simulink subsystem "PipeModule"  (R2021b)
settings: Solver=VariableStepAuto  StartTime=0.0  StopTime=10.0  RelTol=1e-3
libraries: SimscapeFluids_lib x1
settings Model: Creator=silen  LastModifiedBy=silen

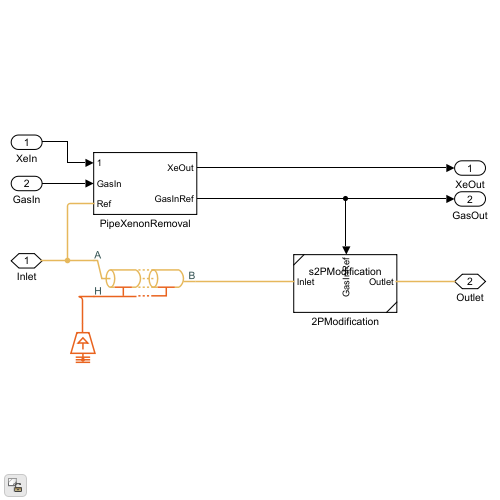
[thumbnail: Simulink's stored preview of the top-level diagram]
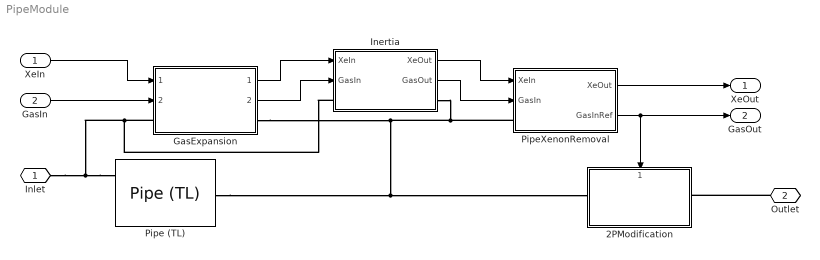
== system PipeModule ==
  XeIn : Inport
  GasIn : Inport  Port=2
  2PModification : Subsystem  ReferencedSubsystem=s2PModification
      settings: PortSchema="{\"entries\":[{\"content\":{\"sides\":[{\"content\":{\"connectorIds\":[\"LConn1\"]},\"type\":\"ConnectorPlacement.EquallySpacedRectSide\",\"uuid\":\"411e3aad-085a-4802-ae1a-063314444375\"},{\"content\":{\"connectorIds\":[\"RConn1\"],\"side\":\"RIGHT\"},\"type\":\"ConnectorPlacement.EquallySpacedRectSide\",\"uuid\":\"fb5502b3-1e9f-42df-a026-3213f778497c\"},{\"content\":{\"connectorIds\":[\"In1\"],\"side\":\"TOP\"},\"type\":\"ConnectorPlacement.EquallySpacedRectSide\",\"uuid\":\"a2632dc0-9484-47d6-bdb2-d7bd34c99042\"}]},\"type\":\"ConnectorPlacement.EquallySpacedConnector\",\"uuid\":\"63fd18a3-6eef-4df0-ac37-70a6f543c0e0\"}],\"packageUris\":[\"http://schema.mathworks.com/mf0/Connector/R2020b\"],\"version\":\"1.0\"}"
  GasExpansion : Subsystem  ReferencedSubsystem=GasExpansion
  Inertia : Subsystem
  Pipe (TL) : SimscapeFluids_lib/Thermal Liquid/Pipes & Fittings/Pipe (TL)  dynamic_compressibility=simscape.enum.onoff.on  inertia=simscape.enum.onoff.off  num_segments=1  pipe_length=5 m  area=0.01 m^2  Dh=0.1128 m  wall_spec=fluids.thermal_liquid.pipes_fittings.enum.wall_spec.rigid  Dh_rigid=0.1128 m  wall_compliance=1.2e-6 m/MPa  wall_time_constant=0.01 s  elevation_spec=foundation.enum.constant_variable.constant  elevation_gain=0 m  g=9.81 m/s^2  pressure_loss_spec=fluids.thermal_liquid.pipes_fittings.enum.PressureLossSpec.Haaland  length_add=1 m  roughness=15e-6 m  Re_friction_TLU=[400, 1000, 1500, 3000, 4000, 6000, 10000, 20000, 40000, 60000, 100000, 100000000]  friction_factor_TLU=[.264, .112, .071, .0417, .0387, .0268, .025, .0232, .0226, .022, .0214, .0214]  shape_factor=64  Re_lam=2000  Re_tur=4000  mdot_nominal=[.1, 1] kg/s  p_diff_nominal=[.001, .01] MPa  mdot_threshold=1e-6 kg/s  heat_transfer_spec=fluids.thermal_liquid.pipes_fittings.enum.HeatTransferSpec.Gnielinski  mdot_nominal_heat=[.1, 1] kg/s  T_in_nominal=[293.15, 293.15] K  T_out_nominal=[300, 300] K  p_in_nominal_heat=[.101325, .101325] MPa  T_wall_nominal=[303.15, 303.15] K  a_coeff=0.023  b_Re_power=0.8  c_Pr_power=0.4  Nu_lam=3.66  Re_Colburn_TLU=[100, 150, 1000]  Colburn_factor_TLU=[.019, .013, .002]  Re_Nu_TLU=[100, 150, 1000]  Pr_Nu_TLU=[1, 10]  Nu_TLU=[3.72, 4.21; 3.75, 4.44; 4.21, 7.15]  T0_vec=293.15 K  p0_vec=0.101325 MPa  mdot0=0.1 kg/s
      settings: SourceProductBaseCode=SH
  PipeXenonRemoval : Subsystem
  Inlet : PMIOPort  Side=Left
  Outlet : PMIOPort  Port=2  Side=Right
  XeOut : Outport
  GasOut : Outport  Port=2
  wires:
  PipeXenonRemoval/1(XeOut) -> XeOut/1
  PipeXenonRemoval/2(GasInRef) -> GasOut/1, 2PModification/1
  XeIn/1 -> GasExpansion/1
  GasIn/1 -> GasExpansion/2
  GasExpansion/1 -> Inertia/1(XeIn)
  GasExpansion/2 -> Inertia/2(GasIn)
  Inertia/2(GasOut) -> PipeXenonRemoval/2(GasIn)
  Inertia/1(XeOut) -> PipeXenonRemoval/1(XeIn)
  connections:
  Pipe (TL)/LConn1 -- Inertia/LConn1 -- GasExpansion/LConn1 -- Inlet/RConn1
  GasExpansion/RConn1 -- PipeXenonRemoval/LConn1 -- Inertia/RConn1 -- 2PModification/LConn1 -- Pipe (TL)/RConn1
  Outlet/RConn1 -- 2PModification/RConn1

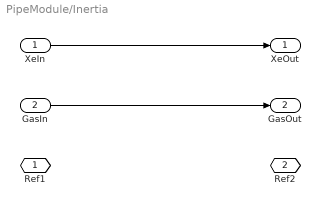
== system PipeModule/Inertia ==
  XeIn : Inport
  GasIn : Inport  Port=2
  Ref1 : PMIOPort  Side=Left
  Ref2 : PMIOPort  Port=2  Side=Right
  XeOut : Outport
  GasOut : Outport  Port=2
  wires:
  XeIn/1 -> XeOut/1
  GasIn/1 -> GasOut/1

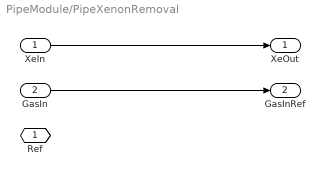
== system PipeModule/PipeXenonRemoval ==
  XeIn : Inport
  GasIn : Inport  Port=2
  Ref : PMIOPort  Side=Left
  XeOut : Outport
  GasInRef : Outport  Port=2
  wires:
  GasIn/1 -> GasInRef/1
  XeIn/1 -> XeOut/1
